simulink model "ziegler_nichols_frekvencijski_sim"  (R2020a)
settings: Solver=FixedStepAuto  StartTime=0.0  StopTime=sim_duration  FixedStep=1e-3  RelTol=1e-3
values from neighbouring files (symbols this model uses):
  C = 470e-6    (= 0.00047)    [linearizacija_simbolicki_script.m]    (also in linearizacija_simbolicki_skripta.m)
  E = 12    [linearizacija_simbolicki_script.m]    (also in linearizacija_simbolicki_skripta.m)
  L = 15.91e-3    (= 0.01591)    [linearizacija_simbolicki_script.m]    (also in linearizacija_simbolicki_skripta.m)
  R = 52    [linearizacija_simbolicki_script.m]    (also in linearizacija_simbolicki_skripta.m)
  ue = eval(ue)    [linearizacija_simbolicki_script.m]    (also in linearizacija_simbolicki_skripta.m)
  x2e = -22.5    [linearizacija_simbolicki_script.m]    (also in linearizacija_simbolicki_skripta.m)
undefined symbols (not defined in the file or in its folder): M, time_step
libraries: powerlib_meascontrol x3
settings Model: Creator=HP  LastModifiedBy=HP

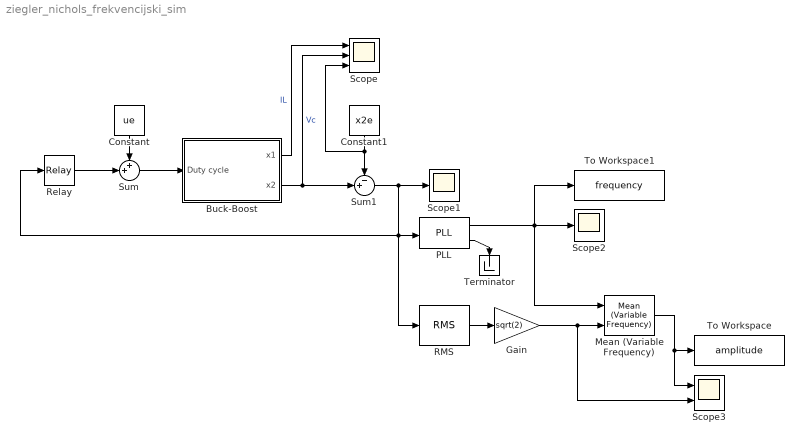
== system ziegler_nichols_frekvencijski_sim ==
  Buck-Boost : Subsystem
  Constant : Constant  Value=ue
  Constant1 : Constant  Value=x2e
  Gain : Gain  Gain=sqrt(2)
  Mean (Variable Frequency) : powerlib_meascontrol/Measurements/Mean (Variable Frequency)  Finit=1  Fmin=1  Vinit=0  Ts=time_step
      settings: SourceProductBaseCode=PS
  PLL : powerlib_meascontrol/PLL/PLL  Fmin=1  Par_Init=[0, 1]  ParK=[180, 3200, 1]  TcD=1e-3  MaxRateChangeFreq=12  FilterCutOffFreq=25  Ts=time_step  AGC=on
      settings: SourceProductBaseCode=PS
  RMS : powerlib_meascontrol/Measurements/RMS  TrueRMS=on  Freq=1  RMSInit=0  Ts=time_step
  Relay : Relay  OffSwitchValue=-eps  OnOutputValue=M  OffOutputValue=-M
  Scope : Scope  NumInputPorts=3
  Scope1 : Scope
  Scope2 : Scope
  Scope3 : Scope  NumInputPorts=2
  Sum : Sum  Inputs=++|
  Sum1 : Sum  Inputs=-+|
  Terminator : Terminator
  To Workspace : ToWorkspace  VariableName=amplitude  SaveFormat=Timeseries  SampleTime=-1
  To Workspace1 : ToWorkspace  VariableName=frequency  SaveFormat=Timeseries  SampleTime=-1
  wires:
  Relay/1 -> Sum/2
  Constant1/1 -> Scope/3, Sum1/1
  Sum1/1 -> Scope1/1, RMS/1, Relay/1, PLL/1
  Constant/1 -> Sum/1
  Buck-Boost/1(x1) -> Scope/1  "IL"
  Sum/1 -> Buck-Boost/1(Duty cycle)
  Buck-Boost/2(x2) -> Sum1/2, Scope/2  "Vc"
  PLL/2 -> Terminator/1
  PLL/1 -> To Workspace1/1, Mean (Variable Frequency)/1, Scope2/1
  Mean (Variable Frequency)/1 -> To Workspace/1, Scope3/1
  RMS/1 -> Gain/1
  Gain/1 -> Scope3/2, Mean (Variable Frequency)/2

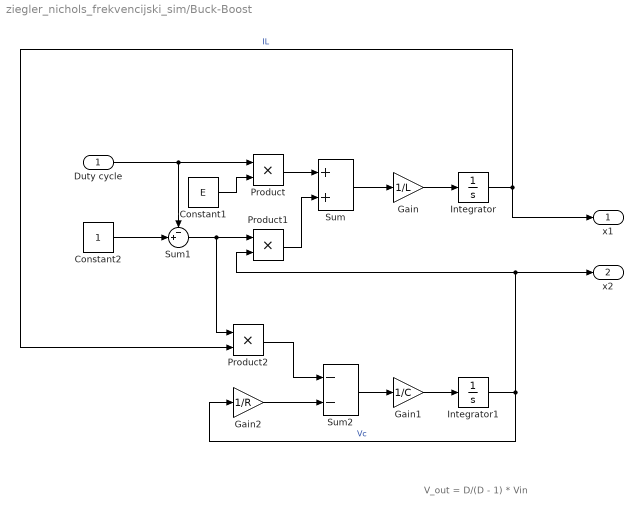
== system ziegler_nichols_frekvencijski_sim/Buck-Boost ==
  note: V_out = D/(D - 1) * Vin
  Duty cycle : Inport
  Constant1 : Constant  Value=E
  Constant2 : Constant
  Gain : Gain  Gain=1/L
  Gain1 : Gain  Gain=1/C
  Gain2 : Gain  Gain=1/R
  Integrator : Integrator
  Integrator1 : Integrator
  Product : Product
  Product1 : Product
  Product2 : Product
  Sum : Sum
  Sum1 : Sum  Inputs=-+|
  Sum2 : Sum  Inputs=--
  x1 : Outport
  x2 : Outport  Port=2
  wires:
  Product/1 -> Sum/1
  Product1/1 -> Sum/2
  Sum2/1 -> Gain1/1
  Constant1/1 -> Product/2
  Integrator1/1 -> Gain2/1, x2/1, Product1/2  "Vc"
  Gain1/1 -> Integrator1/1
  Constant2/1 -> Sum1/2
  Integrator/1 -> x1/1, Product2/2  "IL"
  Sum/1 -> Gain/1
  Gain2/1 -> Sum2/2
  Sum1/1 -> Product2/1, Product1/1
  Duty cycle/1 -> Sum1/1, Product/1
  Product2/1 -> Sum2/1
  Gain/1 -> Integrator/1
